simulink model "fig10_84_Ecoli"  (Simulink 7.9)
settings: Solver=ode45  StartTime=0.0  StopTime=40.0  RelTol=1e-3
settings Model: Creator=Gene Franklin  LastModifiedBy=abbas
settings OptimizationCC: InitFltsAndDblsToZero=on
settings DebuggingCC: SaveWithParameterizedLinksMsg=none  FcnCallInpInsideContextMsg=Use local settings  StrictBusMsg=Warning
settings GRTTargetCC: TargetFcnLib=ansi_tfl_tmw.mat  CombineOutputUpdateFcns=off  GRTInterface=on

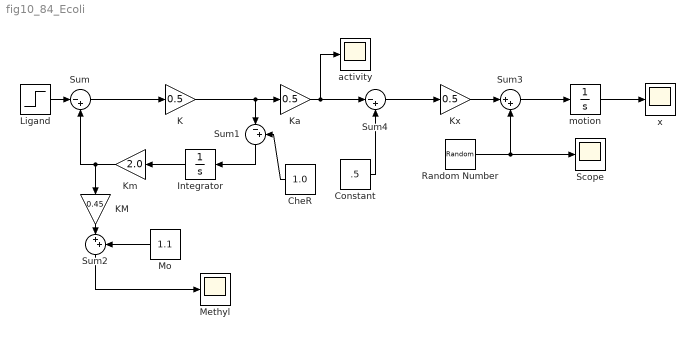
== system fig10_84_Ecoli ==
  CheR : Constant  Value=1.0
  Constant : Constant  Value=.5
  Integrator : Integrator  InitialCondition=1.0
  K : Gain  Gain=0.5
  KM : Gain  Gain=0.45
  Ka : Gain  Gain=0.5
  Km : Gain  Gain=2.0
  Kx : Gain  Gain=0.5
  Ligand : Step  Time=20  After=2.0  SampleTime=0
  Methyl : Scope
      settings: SaveName=EcoliMeth
  Mo : Constant  Value=1.1
  Random Number : RandomNumber  Variance=0.002  SampleTime=0.5
  Scope : Scope
  Sum : Sum  Inputs=|-+
  Sum1 : Sum  Inputs=|-+
  Sum2 : Sum  Inputs=|++
  Sum3 : Sum  Inputs=|++
  Sum4 : Sum  Inputs=|-+
  activity : Scope
      settings: SaveName=EcoliA
  motion : Integrator
  x : Scope
      settings: SaveName=Ecolix
  wires:
  Ligand/1 -> Sum/1
  Sum/1 -> K/1
  Integrator/1 -> Km/1
  Sum1/1 -> Integrator/1
  CheR/1 -> Sum1/2
  K/1 -> Sum1/1, Ka/1
  Km/1 -> Sum/2, KM/1
  Mo/1 -> Sum2/2
  KM/1 -> Sum2/1
  Sum2/1 -> Methyl/1
  motion/1 -> x/1
  Kx/1 -> Sum3/1
  Sum3/1 -> motion/1
  Ka/1 -> Sum4/1, activity/1
  Sum4/1 -> Kx/1
  Constant/1 -> Sum4/2
  Random Number/1 -> Sum3/2, Scope/1
